simulink model "harmonic_oscilator"  (R2017b)
settings: Solver=VariableStepAuto  StartTime=0.0  StopTime=10.0  RelTol=1e-3
undefined symbols (not defined in the file): b, k, m
settings Model: Creator=ASROCK  LastModifiedBy=ASROCK

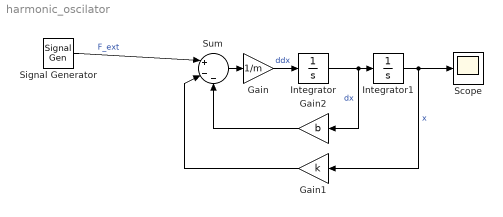
== system harmonic_oscilator ==
  Gain : Gain  Gain=1/m
  Gain1 : Gain  Gain=k
  Gain2 : Gain  Gain=b
  Integrator : Integrator
  Integrator1 : Integrator
  Scope : Scope
  Signal Generator : SignalGenerator  Units=rad/sec
  Sum : Sum  Inputs=|+--
  wires:
  Integrator/1 -> Gain2/1, Integrator1/1  "dx"
  Gain/1 -> Integrator/1  "ddx"
  Signal Generator/1 -> Sum/1  "F_ext"
  Integrator1/1 -> Gain1/1, Scope/1  "x"
  Sum/1 -> Gain/1
  Gain1/1 -> Sum/2
  Gain2/1 -> Sum/3
